simulink model "Lidar_Slam_ROS_Node_R2021a"  (R2021a)
settings: Solver=FixedStepAuto  StartTime=0.0  StopTime=inf  RelTol=1e-3
model workspace (MAT data in the model file):
  SL_ROS_VariableLengthArrays_MaxSizes.CommonInfo.ArrayTruncateAction = 'EmitWarning'
  SL_ROS_VariableLengthArrays_MaxSizes.MsgTypeMap = containers.Map
  SL_ROS_VariableLengthArrays_MaxSizes.MsgTypeMap.serialization.keys = {'sensor_msgs/LaserScan'}
  SL_ROS_VariableLengthArrays_MaxSizes.MsgTypeMap.serialization.values{1}(1).PropertyName = 'Intensities'
  SL_ROS_VariableLengthArrays_MaxSizes.MsgTypeMap.serialization.values{1}(1).DataType = 'single'
  SL_ROS_VariableLengthArrays_MaxSizes.MsgTypeMap.serialization.values{1}(1).MaxLength = 1081
  SL_ROS_VariableLengthArrays_MaxSizes.MsgTypeMap.serialization.values{1}(2).PropertyName = 'Ranges'
  SL_ROS_VariableLengthArrays_MaxSizes.MsgTypeMap.serialization.values{1}(2).DataType = 'single'
  SL_ROS_VariableLengthArrays_MaxSizes.MsgTypeMap.serialization.values{1}(2).MaxLength = 1081
  SL_ROS_VariableLengthArrays_MaxSizes.MsgTypeMap.serialization.uniformity = 0
  SL_ROS_VariableLengthArrays_MaxSizes.MsgTypeMap.serialization.keyType = 'char'
  SL_ROS_VariableLengthArrays_MaxSizes.MsgTypeMap.serialization.valueType = 'any'
undefined symbols (not defined in the file): Theta, X, Y
libraries: robotlib x5, simulink x1
settings Model: Creator=Ron  LastModifiedBy=ZHANG
settings OptimizationCC: EnhancedBackFolding=on  PassReuseOutputArgsAs=Individual arguments  ZeroExternalMemoryAtStartup=off  ZeroInternalMemoryAtStartup=off  MaxStackSize=64  OptimizeBlockOrder=speed  DifferentSizesBufferReuse=on  OptimizationCustomize=off  EfficientTunableParamExpr=on
settings DebuggingCC: ParameterTunabilityLossMsg=error
settings HardwareCC: ProdBitPerPointer=32  ProdBitPerSizeT=32  ProdBitPerPtrDiffT=32  ProdLargestAtomicFloat=None  ProdIntDivRoundTo=Undefined  ProdEndianess=Unspecified  ProdWordSize=32  ProdHWDeviceType=Generic->Unspecified (assume 32-bit Generic)
settings RTWCC: SystemTargetFile=ert.tlc  HardwareBoard=Robot Operating System (ROS)  TLCOptions="-aInlineSetEventsForThisBaseRateFcn=TLC_FALSE -aSuppressMultiTaskScheduler=TLC_FALSE    -aRateBasedStepFcn=0"  TemplateMakefile=ert_default_tmf  Toolchain=Catkin  TargetLang=C++
settings CodeAppCC: ForceParamTrailComments=on  IgnoreCustomStorageClasses=off  OperatorAnnotations=on  SimulinkDataObjDesc=on  SFDataObjDesc=on  InsertBlockDesc=on
settings ERTTargetCC: SupportNonInlinedSFcns=on  SupportVariableSizeSignals=on  ExtModeMexArgs='192.168.80.136' 0 17725  RootIOFormat=Structure reference

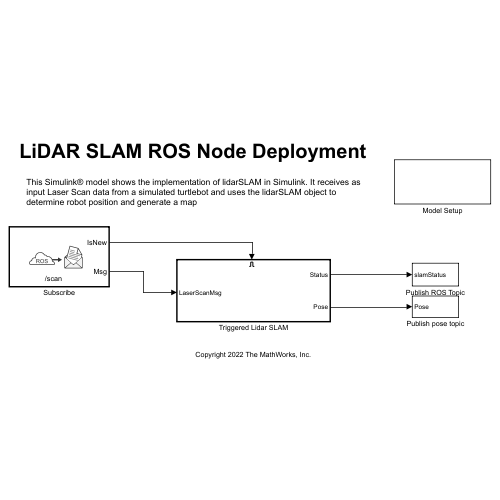
[thumbnail: Simulink's stored preview of the top-level diagram]
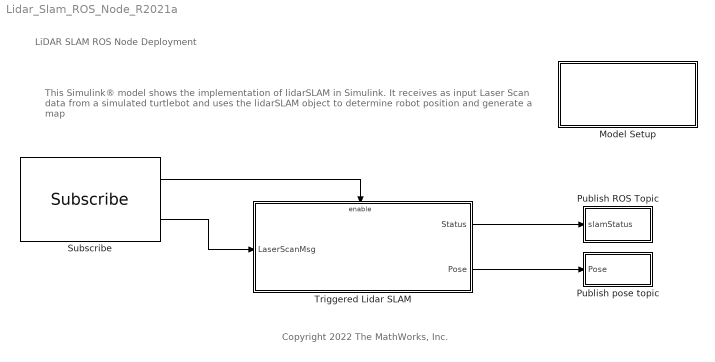
== system Lidar_Slam_ROS_Node_R2021a ==
  note: LiDAR SLAM ROS Node Deployment
  note: This Simulink® model shows the implementation of lidarSLAM in Simulink. It receives as input Laser Scan data from a simulated turtlebot and uses the lidarSLAM object to determine robot position and generate a map
  note: Copyright 2022 The MathWorks, Inc.
  Model Setup : Subsystem
  Publish ROS Topic : Subsystem
  Publish pose topic : Subsystem
  Subscribe : robotlib/Subscribe  topicSource=Select from ROS network  topic=/scan  messageType=sensor_msgs/LaserScan  SampleTime=-1  legacyBusStruct=off  messageQueueLength=1
  Triggered Lidar SLAM : Subsystem
  wires:
  Subscribe/1 -> Triggered Lidar SLAM/Enable
  Subscribe/2 -> Triggered Lidar SLAM/1(LaserScanMsg)
  Triggered Lidar SLAM/1(Status) -> Publish ROS Topic/1(slamStatus)
  Triggered Lidar SLAM/2(Pose) -> Publish pose topic/1(Pose)

== system Lidar_Slam_ROS_Node_R2021a/Model Setup ==
  note: Before running the Simulink model, make sure the ROS network requirements have been set appropriately through the Simulink Toolstrip. Note that setting a Node Host IP address is optional and depends on the computer setup.
  note: ROS Model Setup

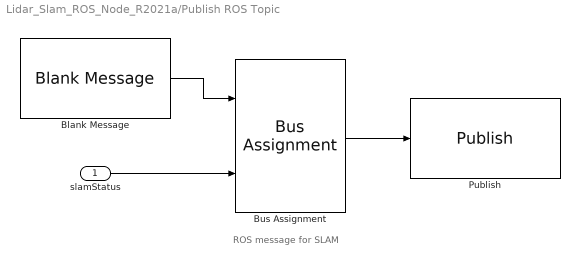
== system Lidar_Slam_ROS_Node_R2021a/Publish ROS Topic ==
  note: ROS message for SLAM
  slamStatus : Inport
  Blank Message : robotlib/Blank Message  messageClass=Message  entityType=std_msgs/Int8  messageType=std_msgs/Int8  SampleTime=inf  legacyBusStruct=off
  Bus Assignment : BusAssignment  AssignedSignals=Data
  Publish : robotlib/Publish  topicSource=Specify your own  topic=/slamStatus  messageType=std_msgs/Int8  legacyBusStruct=off  messageQueueLength=1
  wires:
  Bus Assignment/1 -> Publish/1
  Blank Message/1 -> Bus Assignment/1
  slamStatus/1 -> Bus Assignment/2

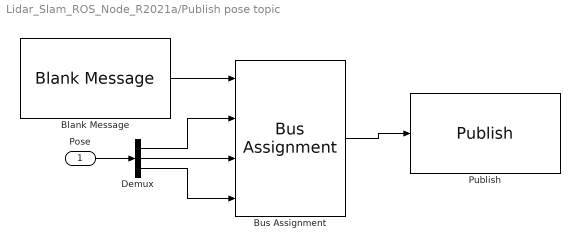
== system Lidar_Slam_ROS_Node_R2021a/Publish pose topic ==
  Pose : Inport
  Blank Message : robotlib/Blank Message  messageClass=Message  entityType=geometry_msgs/Pose2D  messageType=geometry_msgs/Pose2D  SampleTime=inf  legacyBusStruct=off
  Bus Assignment : BusAssignment  AssignedSignals=X,Y,Theta
  Demux : Demux  Outputs=3
  Publish : robotlib/Publish  topicSource=Specify your own  topic=/pose  messageType=geometry_msgs/Pose2D  legacyBusStruct=off  messageQueueLength=1
  wires:
  Blank Message/1 -> Bus Assignment/1
  Bus Assignment/1 -> Publish/1
  Pose/1 -> Demux/1
  Demux/3 -> Bus Assignment/4
  Demux/1 -> Bus Assignment/2
  Demux/2 -> Bus Assignment/3

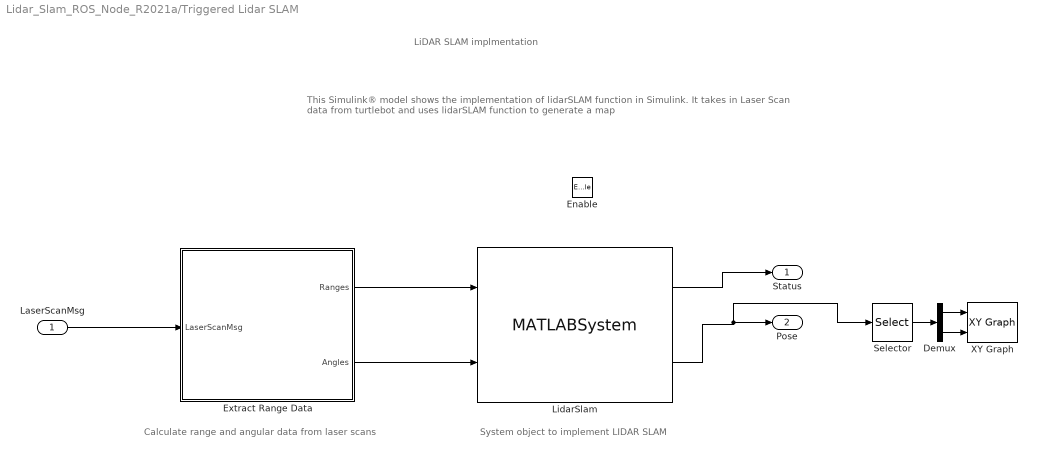
== system Lidar_Slam_ROS_Node_R2021a/Triggered Lidar SLAM ==
  note: Calculate range and angular data from laser scans
  note: LiDAR SLAM implmentation
  note: This Simulink® model shows the implementation of lidarSLAM function in Simulink. It takes in Laser Scan data from turtlebot and uses lidarSLAM function to generate a map
  note: System object to implement LIDAR SLAM
  LaserScanMsg : Inport
  Enable : EnablePort  PropagateVarSize=During execution
  Demux : Demux  Outputs=2
  Extract Range Data : MATLAB Function  TreatAsAtomicUnit=on
  LidarSlam : MATLABSystem  System=LidarSlam  SimulateUsing=Code generation
      mask Type: LidarSlam
      mask Display:
      | disp('LidarSlam');
      | port_label('input',1,'ranges');
      | port_label('input',2,'angles');
      | port_label('output',1,'slamStatus');
      | port_label('output',2,'pose');
  Selector : Selector  InputPortWidth=3  IndexOptions=Index vector (dialog)  Indices=[1 2]  OutputSizes=1
  XY Graph : simulink/Sinks/XY Graph  xmin=-1  xmax=1  ymin=-1  ymax=1  st=-1
  Status : Outport
  Pose : Outport  Port=2
  wires:
  LaserScanMsg/1 -> Extract Range Data/1(LaserScanMsg)
  Extract Range Data/1(Ranges) -> LidarSlam/1
  Extract Range Data/2(Angles) -> LidarSlam/2
  LidarSlam/1 -> Status/1
  LidarSlam/2 -> Pose/1, Selector/1
  Demux/2 -> XY Graph/2
  Demux/1 -> XY Graph/1
  Selector/1 -> Demux/1

== matlab function Lidar_Slam_ROS_Node_R2021a/Triggered Lidar SLAM/Extract Range Data ==
  data: LaserScanMsg input; Ranges output; Angles output
function [Ranges, Angles] = ExtractRangeData(LaserScanMsg)
%#codegen

% Extract Range information
Ranges = double(LaserScanMsg.Ranges);

% Construct Angles vector using AngleMin and AngleIncrement from sensor
% reading.
angMin = double(LaserScanMsg.AngleMin);
angIncrement = double(LaserScanMsg.AngleIncrement);

numReadings = numel(Ranges);
rawAngles = angMin + (0:numReadings-1)' * angIncrement;

% Wrap the angles to the (-pi,pi] interval.
Angles = robotics.internal.wrapToPi(double(rawAngles));
